simulink model "Diode_Clipping_Of_Different_bias_Levels"  (R2014a)
settings: Solver=ode45  StartTime=0.0  StopTime=10.0  RelTol=1e-3
libraries: powerlib x8
settings Model: Creator=mamta  LastModifiedBy=mamta

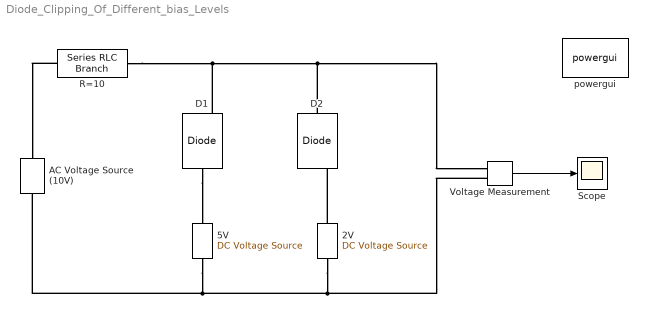
== system Diode_Clipping_Of_Different_bias_Levels ==
  2V : powerlib/Electrical Sources/DC Voltage Source  Amplitude=2  Measurements=None
  5V : powerlib/Electrical Sources/DC Voltage Source  Amplitude=5  Measurements=None
  AC Voltage Source (10V) : powerlib/Electrical Sources/AC Voltage Source  Amplitude=10  Phase=0  Frequency=50  SampleTime=0  Measurements=None
  D1 : powerlib/Power Electronics/Diode  Ron=0.001  Lon=0  Vf=0.8  IC=0  UseSnubber=off  Rs=500  Cs=250e-9  Measurements=on
  D2 : powerlib/Power Electronics/Diode  Ron=0.001  Lon=0  Vf=0.8  IC=0  UseSnubber=off  Rs=500  Cs=250e-9  Measurements=on
  R=10 : powerlib/Elements/Series RLC Branch  LConnTagsString=__new0  RConnTagsString=__new0  BranchType=R  Resistance=10  Inductance=0  SetiL0=off  InitialCurrent=0  Capacitance=1e-6  Setx0=off  InitialVoltage=0  Measurements=None
  Scope : Scope
      settings: YMin=0.8  YMax=0.800003
  Voltage Measurement : powerlib/Measurements/Voltage Measurement  PhasorSimulation=off  OutputType=Complex  PSBequivalent=0
  powergui : powerlib/powergui  Priority=1  SimulationMode=Discrete  SolverType=Tustin  SampleTime=50e-6  frequency=60  SPID=off  DisableSnubberDevices=off  DisableRonSwitches=off  DisableVfSwitches=off  SwTol=0  Interpol=off  DisplayEquations=off  Ts=0  methode=off  frequencyindice=50  Pbase=100e6  ErrMax=1e-4  Iterations=50  UnitsV=kV  UnitsW=MW  FunctionMessages=off  echomessages=off  HookPort=off  EnableUseOfTLC=off  x0status=blocks  RestoreLinks=warning  ResistiveCurrentMeasurement=off  Frange=[0:2:500]  Ylog=off  Xlog=on  ShowGrid=off  save=off  variable=ZData  structure=0  ZoomFFT=off  StartTime=0.0  cycles=1  DisplayStyle=1  fundamental=60  FreqAxis=off  MaxFrequency=1000  frequencyindicesteady=1  RmsSteady=1  display=off
  wires:
  Voltage Measurement/1 -> Scope/1
  connections:
  D1/RConn1 -- Voltage Measurement/LConn1 -- D2/LConn1 -- R=10/RConn1
  AC Voltage Source (10V)/LConn1 -- Voltage Measurement/LConn2 -- 2V/LConn1 -- 5V/RConn1
  R=10/LConn1 -- AC Voltage Source (10V)/RConn1
  D1/LConn1 -- 5V/LConn1
  2V/RConn1 -- D2/RConn1
